simulink library "Pump_Lib"  (R2020b)
settings: Solver=VariableStepAuto  StartTime=0.0  StopTime=10.0  RelTol=1e-3
undefined symbols (not defined in the file): APN_Param
libraries: powerlib x3
Description:
  | Copyright 2019-2020 The MathWorks, Inc.
settings Model: Creator=smiller  LastModifiedBy=smiller
settings SFSimCC: CustomCodeUndefinedFunction=UseInterfaceOnly

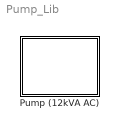
== system Pump_Lib ==
  Pump (12kVA AC) : Subsystem  Variant=on  VariantControlMode=label  LabelModeActiveChoice=Phasor  mask{ModelType=Phasor, PQ_Model=Initial}
      mask prompts: ModelType "Model Type"; PQ_Model "PQ Model"
      mask init:
      | set_param(gcb,'LabelModeActiveChoice',get_param(gcb,'ModelType'));
      | set_param([gcb '/Phasor'],'PQ_Model',get_param(gcb,'PQ_Model'));
      settings: AttributesFormatString=%<BlockChoice>
      mask TypeOptions ModelType: Detailed | Phasor
      mask TypeOptions PQ_Model: Initial | Tuned
      mask Display:
      | blk=find_system(gcbh, 'SearchDepth', 1,'FollowLinks','on','LookUnderMasks','all', 'Parent', gcb,'VariantObject', get_param(gcb,'activevariant'));
      | eval(get_param(blk, 'MaskDisplay'));

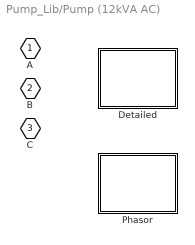
== system Pump_Lib/Pump (12kVA AC) ==
  Detailed : Subsystem  VariantControl=Detailed
      mask Display: image('PumpAC_Detailed_IMAGE.jpg');
  Phasor : Subsystem  VariantControl=Phasor  mask{PQ_Model=Initial}
      mask prompts: PQ_Model "PQ Model"
      mask init:
      | set_param([gcb '/Calc PQ'],'PQ_Model',get_param(gcb,'PQ_Model'));
      mask TypeOptions PQ_Model: Initial | Tuned
      mask Display: image('PumpAC_Phasor_IMAGE.jpg');
  A : PMIOPort  Side=Left
  B : PMIOPort  Port=2  Side=Left
  C : PMIOPort  Port=3  Side=Left

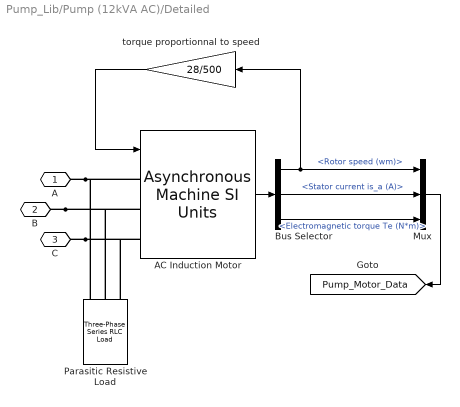
== system Pump_Lib/Pump (12kVA AC)/Detailed ==
  AC Induction Motor : powerlib/Machines/Asynchronous Machine SI Units  RotorType=Squirrel-cage  PresetModel=No  MechanicalLoad=Torque Tm  ShowDetailedParameters=on  ReferenceFrame=Rotor  Units=SI  MeasurementBus=off  NominalParameters=[12e3 200 400]  Stator=[0.2761 0.002191/10]  Rotor=[0.16 0.002191/10]  Cage1=[ 0.022 0.226/377]  Cage2=[ 0.022 0.226/377]  Lm=0.07614  Mechanical=[0.01 0 8]  PolePairs=8  InitialConditions=[0 0 0.850924 0.850924 0.850924 -89.9171 -209.917 30.0829]*0+[0,0 0,0,0 0,0,0]  SimulateSaturation=off  Saturation=[14.03593122, 27.81365428, 53.79336849, 72.68890987, 97.98006896, 148.6815601, 215.7428561, 302.9841135, 428.7778367 ; 230, 322, 414, 460, 506, 552, 598, 644, 690]  LoadFlowParameters=0  TsPowergui=0  TsBlock=-1  IterativeModel=Forward Euler  IterativeDiscreteModel=Trapezoidal non iterative  Pmec=0
  Bus Selector : BusSelector  OutputSignals=Mechanical.Rotor speed (wm),Stator measurements.Stator current is_a (A),Mechanical.Electromagnetic torque Te (N*m)
  Mux : Mux  Inputs=3
  Parasitic Resistive Load : powerlib/Elements/Three-Phase Series RLC Load  LConnTagsString=A|B|C  Configuration=Y (grounded)  NominalVoltage=200  Vabc=[1e3 1e3 1e3]  Vabcp=[1e3 1e3 1e3]  NominalFrequency=400  UnbalancedPower=off  ActivePower=1200  InductivePower=0  CapacitivePower=0  Pabc=[10e3 9e3 11e3]  QLabc=[100 90 110]  QCabc=[100 90 110]  Pabcp=[10e3 9e3 11e3]  QLabcp=[100 90 110]  QCabcp=[100 90 110]  Measurements=None  LoadType=constant Z
  torque proportionnal to speed : Gain  Gain=28/500
  A : PMIOPort  Side=Left
  B : PMIOPort  Port=2  Side=Left
  C : PMIOPort  Port=3  Side=Left
  tag scope: Pump_Motor_Data=global
  wires:
  Mux/1 -> [Pump_Motor_Data]
  AC Induction Motor/1 -> Bus Selector/1
  Bus Selector/1 -> torque proportionnal to speed/1, Mux/1  "<Rotor speed (wm)>"
  torque proportionnal to speed/1 -> AC Induction Motor/1
  Bus Selector/2 -> Mux/2  "<Stator current is_a (A)>"
  Bus Selector/3 -> Mux/3  "<Electromagnetic torque Te (N*m)>"
  connections:
  B/RConn1 -- Parasitic Resistive Load/LConn2 -- AC Induction Motor/LConn2
  A/RConn1 -- Parasitic Resistive Load/LConn1 -- AC Induction Motor/LConn1
  C/RConn1 -- Parasitic Resistive Load/LConn3 -- AC Induction Motor/LConn3

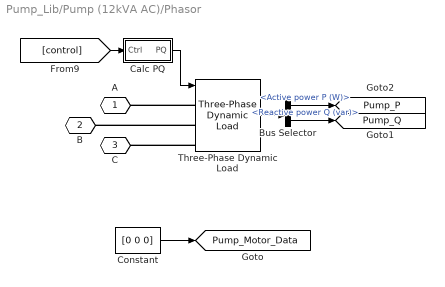
== system Pump_Lib/Pump (12kVA AC)/Phasor ==
  Bus Selector : BusSelector  OutputSignals=Active power P (W),Reactive power Q (var)
  Calc PQ : Subsystem  Variant=on  VariantControlMode=label  LabelModeActiveChoice=Initial  mask{PQ_Model=Initial}
      mask prompts: PQ_Model "PQ Model"
      mask init:
      | set_param(gcb,'LabelModeActiveChoice',get_param(gcb,'PQ_Model'));
      settings: AttributesFormatString=%<BlockChoice>
      mask TypeOptions PQ_Model: Initial | Tuned
      mask Display: disp(' ')
  Constant : Constant  Value=[0 0 0]
  Three-Phase Dynamic Load : powerlib/Elements/Three-Phase Dynamic Load  NominalVoltage=[ 500e3 400 ]  ActiveReactivePowers=[APN_Param.Pump.P APN_Param.Pump.Q]  PositiveSequence=[0.0004 0]  ExternalControl=on  NpNq=[1.3 2]  TimeConstants="[0  0  0  0]"  MinimumVoltage=0.7  Tfilter=1e-4  LoadFlowParameters=[4 0 0 0 0]
      settings: SourceProductBaseCode=PS
  A : PMIOPort  Side=Left
  B : PMIOPort  Port=2  Side=Left
  C : PMIOPort  Port=3  Side=Left
  tag scope: Pump_Motor_Data=global, Pump_P=global, Pump_Q=global
  wires:
  Constant/1 -> [Pump_Motor_Data]
  Calc PQ/1(PQ) -> Three-Phase Dynamic Load/1
  [control] -> Calc PQ/1(Ctrl)
  Bus Selector/2 -> [Pump_Q]  "<Reactive power Q (var)>"
  Three-Phase Dynamic Load/1 -> Bus Selector/1
  Bus Selector/1 -> [Pump_P]  "<Active power P (W)>"
  connections:
  Three-Phase Dynamic Load/LConn1 -- A/RConn1
  Three-Phase Dynamic Load/LConn2 -- B/RConn1
  Three-Phase Dynamic Load/LConn3 -- C/RConn1

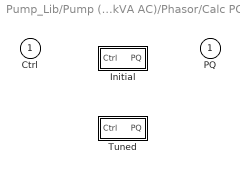
== system Pump_Lib/Pump (12kVA AC)/Phasor/Calc PQ ==
  Ctrl : Inport
  Initial : Subsystem  VariantControl=Initial
  Tuned : Subsystem  VariantControl=Tuned
  PQ : Outport  VectorParamsAs1DForOutWhenUnconnected=off

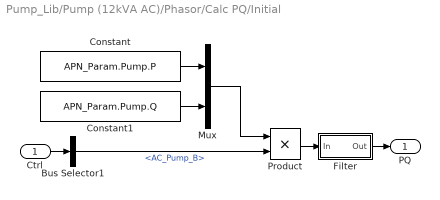
== system Pump_Lib/Pump (12kVA AC)/Phasor/Calc PQ/Initial ==
  Ctrl : Inport
  Bus Selector1 : BusSelector  OutputSignals=AC_Pump_B
  Constant : Constant  Value=APN_Param.Pump.P
  Constant1 : Constant  Value=APN_Param.Pump.Q
  Filter : Subsystem  mask(First-order lag supporting vector signals){b=1e-2, x_initial=[APN_Param.Pump.P APN_Param.Pump.Q]*0}
      mask prompts: b "Filter time constant"; x_initial "Initial output"
      mask help: Models a lag of the form 1/(b*s+1) where s is the Laplace operator.
  Mux : Mux  Inputs=2
  Product : Product
  PQ : Outport  VectorParamsAs1DForOutWhenUnconnected=off
  wires:
  Constant1/1 -> Mux/2
  Constant/1 -> Mux/1
  Ctrl/1 -> Bus Selector1/1
  Mux/1 -> Product/1
  Bus Selector1/1 -> Product/2  "<AC_Pump_B>"
  Filter/1(Out) -> PQ/1
  Product/1 -> Filter/1(In)

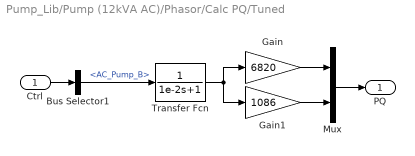
== system Pump_Lib/Pump (12kVA AC)/Phasor/Calc PQ/Tuned ==
  Ctrl : Inport
  Bus Selector1 : BusSelector  OutputSignals=AC_Pump_B
  Gain : Gain  Gain=6820
  Gain1 : Gain  Gain=1086
  Mux : Mux  Inputs=2
  Transfer Fcn : TransferFcn  Denominator=[1e-2 1]
  PQ : Outport  VectorParamsAs1DForOutWhenUnconnected=off
  wires:
  Transfer Fcn/1 -> Gain1/1, Gain/1
  Mux/1 -> PQ/1
  Gain/1 -> Mux/1
  Gain1/1 -> Mux/2
  Bus Selector1/1 -> Transfer Fcn/1  "<AC_Pump_B>"
  Ctrl/1 -> Bus Selector1/1

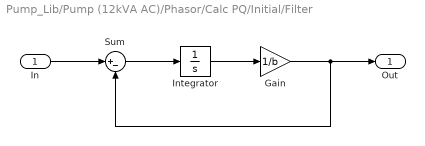
== system Pump_Lib/Pump (12kVA AC)/Phasor/Calc PQ/Initial/Filter ==
  In : Inport
  Gain : Gain  Gain=1/b
  Integrator : Integrator  InitialCondition=x_initial
  Sum : Sum  Inputs=|+-  InputSameDT=on  SaturateOnIntegerOverflow=on  OutDataTypeStr=Inherit: Same as first input
  Out : Outport  VectorParamsAs1DForOutWhenUnconnected=off
  wires:
  Sum/1 -> Integrator/1
  In/1 -> Sum/1
  Integrator/1 -> Gain/1
  Gain/1 -> Sum/2, Out/1
